simulink model "q_ip02_position"  (R2022b)
settings: Solver=ode4  StartTime=0.0  StopTime=5*60  FixedStep=0.002  RelTol=1e-3  AbsTol=1e-6  EnableMultiTasking=on
undefined symbols (not defined in the file): HIL, K, K_AMP, K_EC, K_EP, kp, kv, qc_get_step_size, tau, VMAX_AMP, VMAX_DAC, wcf, X_LIM_ENABLE, X_MAX, X_MIN, zetaf
libraries: quarc_library x5, simulink_extras x1
settings Model: SimulationMode=external  ExtModeTrigDuration=10000  Creator=Mfotoohi  LastModifiedBy=tst2753
settings SolverCC: AutoScaleAbsTol=off  AlgebraicLoopSolver=TrustRegion  PositivePriorityOrder=on
settings DataIOCC: SaveFormat=Array  SignalLoggingSaveFormat=ModelDataLogs  ReturnWorkspaceOutputs=off
settings OptimizationCC: BooleanDataType=off  OptimizeBlockIOStorage=off  BufferReuse=off  ExpressionFolding=off  ExpressionDepthLimit=2147483647  LocalBlockOutputs=off  InitFltsAndDblsToZero=on
settings DebuggingCC: SaveWithParameterizedLinksMsg=none  UnderspecifiedInitializationDetection=Classic  MergeDetectMultiDrivingBlocksExec=none  SignalResolutionControl=TryResolveAllWithWarning  MultiTaskDSMMsg=warning  MultiTaskCondExecSysMsg=none  FcnCallInpInsideContextMsg=warning  UnconnectedInputMsg=warning  UnconnectedOutputMsg=warning  UnconnectedLineMsg=warning  StateNameClashWarn=warning  SFUnexpectedBacktrackingDiag=warning  SFNoUnconditionalDefaultTransitionDiag=warning  SFExecutionAtInitializationDiag=none  SFMachineParentedDataDiag=warning  ArithmeticOperatorsInVariantConditions=warning
settings HardwareCC: ProdBitPerPointer=32  ProdBitPerSizeT=32  ProdBitPerPtrDiffT=32  ProdWordSize=32  ProdHWDeviceType=Intel->x86-32 (Windows32)  TargetHWDeviceType=32-bit Generic
settings ModelReferenceCC: PropagateSignalLabelsOutOfModel=off
settings SFSimCC: SimUseLocalCustomCode=off  CustomCodeUndefinedFunction=UseInterfaceOnly
settings RTWCC: Description=QUARC Win32 Target Using Toolchain  SystemTargetFile=quarc_windows.tlc  TemplateMakefile=quarc_default_tmf  RTWUseLocalCustomCode=off  Toolchain=QUARC windows | nmake (64-bit Windows)  BuildConfiguration=Faster Runs
settings CodeAppCC: StateflowObjectComments=on
settings STFCustomTargetCC: ConcurrentExecutionCompliant=on  GRTInterface=on  UseToolchainInfoCompliant=on  SystemTargetFile=quarc_windows.tlc
settings GRTTargetCC: TargetLangStandard=C89/C90 (ANSI)  ParMdlRefBuildCompliant=off  CompOptLevelCompliant=off  CombineOutputUpdateFcns=off  MatFileLogging=off  CPPClassGenCompliant=off  GRTInterface=on  ExtMode=on  ExtModeMexFile=quarc_comm
settings ConfigComp: CovMetricSettings=dw  CovSaveCumulativeToWorkspaceVar=on  CovSaveSingleToWorkspaceVar=on  CovExternalEMLEnable=off

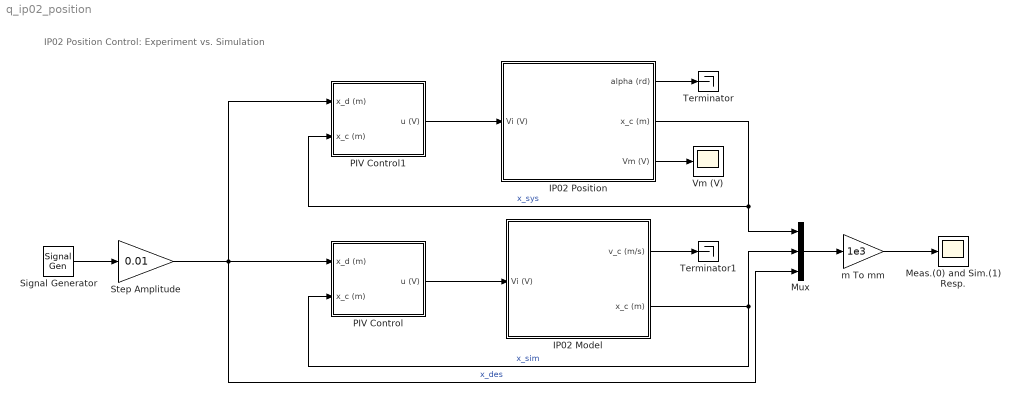
== system q_ip02_position ==
  note: IP02 Position Control:
      | Experiment vs. Simulation
  IP02 Model : Subsystem
  IP02 Position : Subsystem
  Meas.(0) and Sim.(1) Resp. : Scope
  Mux : Mux  Inputs=3
  PIV Control : Subsystem
  PIV Control1 : Subsystem
  Signal Generator : SignalGenerator  WaveForm=square  Frequency=0.66
  Step Amplitude : Gain  Gain=0.01  SaturateOnIntegerOverflow=on  OutDataTypeStr=Inherit: Same as input  ParamDataTypeStr=Inherit: Same as input
  Terminator : Terminator
  Terminator1 : Terminator
  Vm (V) : Scope
  m To mm : Gain  Gain=1e3  SaturateOnIntegerOverflow=on  OutDataTypeStr=Inherit: Same as input  ParamDataTypeStr=Inherit: Same as input
  wires:
  IP02 Model/2(x_c (m)) -> PIV Control/2(x_c (m)), Mux/2  "x_sim"
  Mux/1 -> m To mm/1
  m To mm/1 -> Meas.(0) and Sim.(1) Resp./1
  Signal Generator/1 -> Step Amplitude/1
  Step Amplitude/1 -> PIV Control1/1(x_d (m)), Mux/3, PIV Control/1(x_d (m))  "x_des"
  PIV Control/1(u (V)) -> IP02 Model/1(Vi (V))
  PIV Control1/1(u (V)) -> IP02 Position/1(Vi (V))
  IP02 Position/1(alpha (rd)) -> Terminator/1
  IP02 Position/3(Vm (V)) -> Vm (V)/1
  IP02 Position/2(x_c (m)) -> Mux/1, PIV Control1/2(x_c (m))  "x_sys"
  IP02 Model/1(v_c (m/s)) -> Terminator1/1

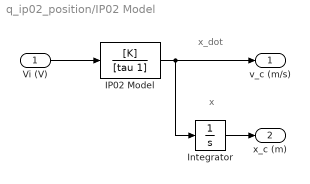
== system q_ip02_position/IP02 Model ==
  note: x_dot
  note: x
  Vi (V) : Inport
  IP02 Model : TransferFcn  Numerator=[K]  Denominator=[tau 1]
  Integrator : Integrator
  v_c (m/s) : Outport
  x_c (m) : Outport  Port=2
  wires:
  IP02 Model/1 -> v_c (m/s)/1, Integrator/1
  Vi (V)/1 -> IP02 Model/1
  Integrator/1 -> x_c (m)/1

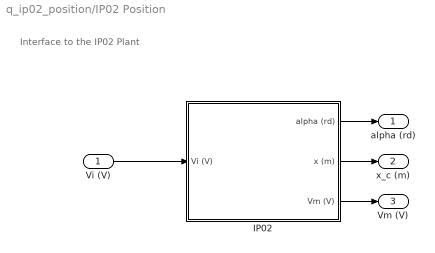
== system q_ip02_position/IP02 Position ==
  note: Interface to the IP02 Plant
  Vi (V) : Inport
  IP02 : Subsystem
  alpha (rd) : Outport  InitialOutput=0
  x_c (m) : Outport  Port=2  InitialOutput=0
  Vm (V) : Outport  Port=3  InitialOutput=0
  wires:
  IP02/3(Vm (V)) -> Vm (V)/1
  Vi (V)/1 -> IP02/1(Vi (V))
  IP02/1(alpha (rd)) -> alpha (rd)/1
  IP02/2(x (m)) -> x_c (m)/1

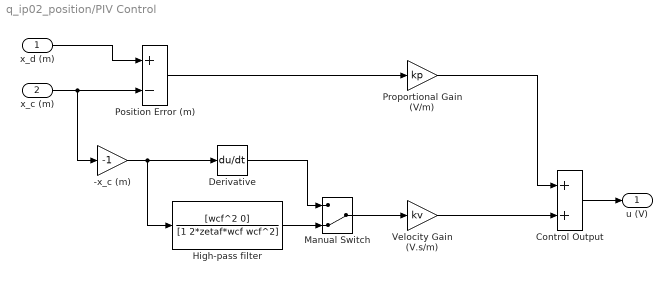
== system q_ip02_position/PIV Control ==
  x_d (m) : Inport
  x_c (m) : Inport  Port=2
  -x_c (m) : Gain  Gain=-1
  Control Output : Sum
  Derivative : Derivative
  High-pass filter : TransferFcn  Numerator=[wcf^2 0]  Denominator=[1 2*zetaf*wcf wcf^2]
  Manual Switch : ManualSwitch  CurrentSetting=0
  Position Error (m) : Sum  Inputs=+-
  Proportional Gain (V/m) : Gain  Gain=kp
  Velocity Gain (V.s/m) : Gain  Gain=kv
  u (V) : Outport
  wires:
  Proportional Gain (V/m)/1 -> Control Output/1
  x_d (m)/1 -> Position Error (m)/1
  Control Output/1 -> u (V)/1
  x_c (m)/1 -> Position Error (m)/2, -x_c (m)/1
  Position Error (m)/1 -> Proportional Gain (V/m)/1
  -x_c (m)/1 -> Derivative/1, High-pass filter/1
  High-pass filter/1 -> Manual Switch/2
  Manual Switch/1 -> Velocity Gain (V.s/m)/1
  Derivative/1 -> Manual Switch/1
  Velocity Gain (V.s/m)/1 -> Control Output/2

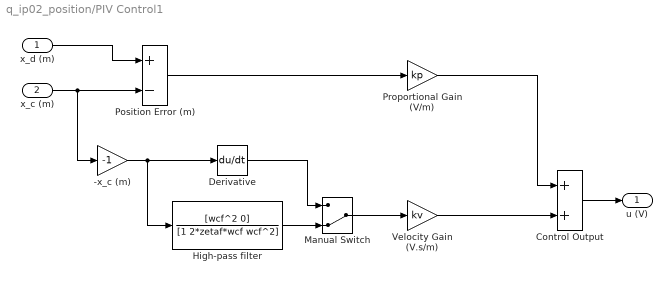
== system q_ip02_position/PIV Control1 ==
  x_d (m) : Inport
  x_c (m) : Inport  Port=2
  -x_c (m) : Gain  Gain=-1
  Control Output : Sum
  Derivative : Derivative
  High-pass filter : TransferFcn  Numerator=[wcf^2 0]  Denominator=[1 2*zetaf*wcf wcf^2]
  Manual Switch : ManualSwitch  CurrentSetting=0
  Position Error (m) : Sum  Inputs=+-
  Proportional Gain (V/m) : Gain  Gain=kp
  Velocity Gain (V.s/m) : Gain  Gain=kv
  u (V) : Outport
  wires:
  Proportional Gain (V/m)/1 -> Control Output/1
  x_d (m)/1 -> Position Error (m)/1
  Control Output/1 -> u (V)/1
  x_c (m)/1 -> Position Error (m)/2, -x_c (m)/1
  Position Error (m)/1 -> Proportional Gain (V/m)/1
  -x_c (m)/1 -> Derivative/1, High-pass filter/1
  High-pass filter/1 -> Manual Switch/2
  Manual Switch/1 -> Velocity Gain (V.s/m)/1
  Derivative/1 -> Manual Switch/1
  Velocity Gain (V.s/m)/1 -> Control Output/2

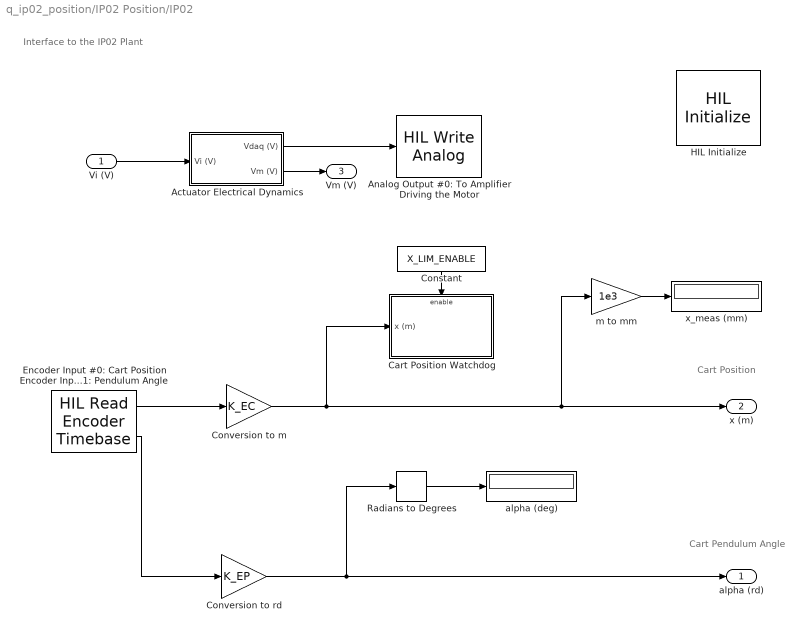
== system q_ip02_position/IP02 Position/IP02 ==
  note: Cart Pendulum Angle
  note: Cart Position
  note: Interface to the IP02 Plant
  Vi (V) : Inport
  Actuator Electrical Dynamics : Subsystem
  Analog Output #0: To Amplifier Driving the Motor : quarc_library/Data Acquisition/Generic/Immediate I//O/HIL Write Analog  Tag=unassigned  object_name=HIL-1  channels=0  sample_time=-1  active=on  vector_input=on
  Cart Position Watchdog : Subsystem  TreatAsAtomicUnit=on
  Constant : Constant  Value=X_LIM_ENABLE
  Conversion to m : Gain  Gain=K_EC  SaturateOnIntegerOverflow=on  OutDataTypeStr=Inherit: Same as input  ParamDataTypeStr=Inherit: Same as input
  Conversion to rd : Gain  Gain=K_EP  SaturateOnIntegerOverflow=on  OutDataTypeStr=Inherit: Same as input  ParamDataTypeStr=Inherit: Same as input
  Encoder Input #0: Cart Position Encoder Input #1: Pendulum Angle : quarc_library/Data Acquisition/Generic/Timebases/HIL Read Encoder Timebase  Tag=unassigned  object_name=HIL-1  clock=0  channels=[0,1]  active=on  vector_output=off  data_type_mode=Inherit via back propagation  data_type=double  overflow_mode=Error on overflow  samples_in_buffer=max(ceil(1/qc_get_step_size), 1)
  HIL Initialize : quarc_library/Data Acquisition/Generic/Configuration/HIL Initialize  object_name=HIL-1  board_type=q2_usb  board_number=0  board_options=d0=digital;d1=digital;led=auto;update_rate=normal;decimation=1  exclusive=off  active=off  hardware_clocks=[0:2]  clock_modes=[]  initial_clock_frequencies=[]  set_clock_params_at_start=off  set_clock_params_at_switch_in=off  set_clock_frequencies_at_start=off  set_clock_frequencies_at_switch_in=off  analog_input_channels=[0:1]  analog_input_configurations=[]  analog_input_maximums=10  analog_input_minimums=-10  set_analog_input_params_at_start=on  set_analog_input_params_at_switch_in=off  analog_output_channels=[0:1]  analog_output_maximums=10  analog_output_minimums=-10  initial_analog_outputs=[0]  final_analog_outputs=[0]  watchdog_analog_outputs=0  set_analog_output_params_at_start=on  set_analog_output_params_at_switch_in=off  set_analog_outputs_at_start=on  set_analog_outputs_at_switch_in=off  set_analog_outputs_at_terminate=on  set_analog_outputs_at_switch_out=off  set_analog_outputs_on_watchdog=off  digital_input_channels=[]  digital_output_channels=[]  digital_output_configuration=[]  initial_digital_outputs=[1]  final_digital_outputs=[1]  watchdog_digital_outputs=[1]  set_digital_output_params_at_start=off  set_digital_output_params_at_switch_in=off  set_digital_outputs_at_start=on  set_digital_outputs_at_switch_in=off  set_digital_outputs_at_terminate=on  set_digital_outputs_at_switch_out=off  set_digital_outputs_on_watchdog=off  encoder_channels=[0:1]  quadrature=[4]  encoder_filter_frequency=[]  initial_encoder_counts=[0]  set_encoder_params_at_start=on  set_encoder_params_at_switch_in=off  set_encoder_counts_at_start=on  set_encoder_counts_at_switch_in=off  pwm_channels=[]  pwm_modes=[0]  pwm_frequency=1/0.020  pwm_configuration=[]  pwm_alignment=[]  pwm_polarity=[]  pwm_leading_deadband=[]  pwm_trailing_deadband=[]  initial_pwm_outputs=[0]  final_pwm_outputs=[0]  watchdog_pwm_outputs=[0]  set_pwm_params_at_start=on  set_pwm_params_at_switch_in=off  set_pwm_outputs_at_start=on  set_pwm_outputs_at_switch_in=off  set_pwm_outputs_at_terminate=on  set_pwm_outputs_at_switch_out=off  set_pwm_outputs_on_watchdog=off  other_output_channels=[]  initial_other_outputs=[]  final_other_outputs=[]  watchdog_other_outputs=[]  set_other_outputs_at_start=off  set_other_outputs_at_switch_in=off  set_other_outputs_at_terminate=off  set_other_outputs_at_switch_out=off  set_other_outputs_on_watchdog=off
  Radians to Degrees : simulink_extras/Transformations/Radians to Degrees
  alpha (deg) : Display
      settings: Decimation=100
  m to mm : Gain  Gain=1e3  SaturateOnIntegerOverflow=on  OutDataTypeStr=Inherit: Same as input  ParamDataTypeStr=Inherit: Same as input
  x_meas (mm) : Display
      settings: Decimation=100
  alpha (rd) : Outport  InitialOutput=0
  x (m) : Outport  Port=2  InitialOutput=0
  Vm (V) : Outport  Port=3  InitialOutput=0
  wires:
  Encoder Input #0: Cart Position Encoder Input #1: Pendulum Angle/1 -> Conversion to m/1
  Conversion to m/1 -> Cart Position Watchdog/1(x (m)), x (m)/1, m to mm/1
  m to mm/1 -> x_meas (mm)/1
  Encoder Input #0: Cart Position Encoder Input #1: Pendulum Angle/2 -> Conversion to rd/1
  Radians to Degrees/1 -> alpha (deg)/1
  Conversion to rd/1 -> Radians to Degrees/1, alpha (rd)/1
  Constant/1 -> Cart Position Watchdog/Enable
  Actuator Electrical Dynamics/1(Vdaq (V)) -> Analog Output #0: To Amplifier Driving the Motor/1
  Vi (V)/1 -> Actuator Electrical Dynamics/1(Vi (V))
  Actuator Electrical Dynamics/2(Vm (V)) -> Vm (V)/1

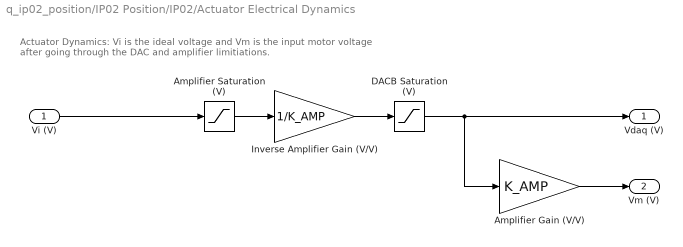
== system q_ip02_position/IP02 Position/IP02/Actuator Electrical Dynamics ==
  note: Actuator Dynamics: Vi is the ideal voltage and Vm is the
      | input motor voltage after going through the DAC and amplifier limitiations.
  Vi (V) : Inport
  Amplifier Gain (V/V) : Gain  Gain=K_AMP
  Amplifier Saturation (V) : Saturate  UpperLimit=VMAX_AMP  LowerLimit=-VMAX_AMP
  DACB Saturation (V) : Saturate  UpperLimit=VMAX_DAC  LowerLimit=-VMAX_DAC
  Inverse Amplifier Gain (V/V) : Gain  Gain=1/K_AMP
  Vdaq (V) : Outport
  Vm (V) : Outport  Port=2
  wires:
  Vi (V)/1 -> Amplifier Saturation (V)/1
  Amplifier Saturation (V)/1 -> Inverse Amplifier Gain (V/V)/1
  Inverse Amplifier Gain (V/V)/1 -> DACB Saturation (V)/1
  DACB Saturation (V)/1 -> Amplifier Gain (V/V)/1, Vdaq (V)/1
  Amplifier Gain (V/V)/1 -> Vm (V)/1

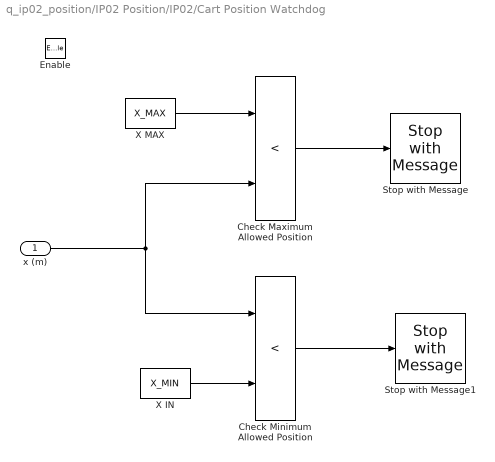
== system q_ip02_position/IP02 Position/IP02/Cart Position Watchdog ==
  x (m) : Inport
  Enable : EnablePort
  Check Maximum Allowed Position : RelationalOperator  Operator=<
  Check Minimum Allowed Position : RelationalOperator  Operator=<
  Stop with Message : quarc_library/Sinks/Error Handling/Stop with Message  message_type=Fixed error message  message_icon=Error  message=Maximum Limit Reached.
  Stop with Message1 : quarc_library/Sinks/Error Handling/Stop with Message  message_type=Fixed error message  message_icon=Error  message=Minimum Limit Reached.
  X IN : Constant  Value=X_MIN
  X MAX : Constant  Value=X_MAX
  wires:
  Check Maximum Allowed Position/1 -> Stop with Message/1
  x (m)/1 -> Check Minimum Allowed Position/1, Check Maximum Allowed Position/2
  X IN/1 -> Check Minimum Allowed Position/2
  Check Minimum Allowed Position/1 -> Stop with Message1/1
  X MAX/1 -> Check Maximum Allowed Position/1
